simulink model "Channel"  (R2023b)
settings: Solver=VariableStepAuto  StartTime=0.0  StopTime=0.01  MaxStep=1e-3  RelTol=1e-3
libraries: simulink x6, dspsrcs4 x1, dspsigops x1
(part 2 of 3)

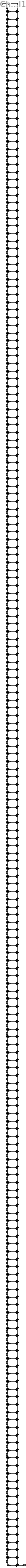
== system Channel/Digital Telecom Project Channel1 ==
  Input : Inport
  BodyDelay{3..205} (203 alike) : Delay  DelayLength=1  InitialCondition=0
  BodyDelay2 : Delay  DelayLength=1  InitialCondition=0  SampleTime=1e-5
  BodyLSum{2..205} (204 alike) : Sum  Inputs=++|  RndMeth=Nearest  SaturateOnIntegerOverflow=on  OutDataTypeStr=Inherit: Same as first input
  b(1) : Gain  Gain=-7.23177798125752776e-05  ParamDataTypeStr=double  RndMeth=Nearest  SaturateOnIntegerOverflow=on  OutDataTypeStr=Inherit: Same as input
  b(10) : Gain  Gain=-0.00017738558129430735  ParamDataTypeStr=double  RndMeth=Nearest  SaturateOnIntegerOverflow=on  OutDataTypeStr=Inherit: Same as input
  b(100) : Gain  Gain=0.0554462164918697528  ParamDataTypeStr=double  RndMeth=Nearest  SaturateOnIntegerOverflow=on  OutDataTypeStr=Inherit: Same as input
  b(101) : Gain  Gain=0.0571275400140215384  ParamDataTypeStr=double  RndMeth=Nearest  SaturateOnIntegerOverflow=on  OutDataTypeStr=Inherit: Same as input
  b(102) : Gain  Gain=0.0581515970344804387  ParamDataTypeStr=double  RndMeth=Nearest  SaturateOnIntegerOverflow=on  OutDataTypeStr=Inherit: Same as input
  b(103) : Gain  Gain=0.0584955166074403385  ParamDataTypeStr=double  RndMeth=Nearest  SaturateOnIntegerOverflow=on  OutDataTypeStr=Inherit: Same as input
  b(104) : Gain  Gain=0.0581515970344804387  ParamDataTypeStr=double  RndMeth=Nearest  SaturateOnIntegerOverflow=on  OutDataTypeStr=Inherit: Same as input
  b(105) : Gain  Gain=0.0571275400140215384  ParamDataTypeStr=double  RndMeth=Nearest  SaturateOnIntegerOverflow=on  OutDataTypeStr=Inherit: Same as input
  b(106) : Gain  Gain=0.0554462164918697528  ParamDataTypeStr=double  RndMeth=Nearest  SaturateOnIntegerOverflow=on  OutDataTypeStr=Inherit: Same as input
  b(107) : Gain  Gain=0.0531450506077565596  ParamDataTypeStr=double  RndMeth=Nearest  SaturateOnIntegerOverflow=on  OutDataTypeStr=Inherit: Same as input
  b(108) : Gain  Gain=0.0502749556371871673  ParamDataTypeStr=double  RndMeth=Nearest  SaturateOnIntegerOverflow=on  OutDataTypeStr=Inherit: Same as input
  b(109) : Gain  Gain=0.0468989161408221791  ParamDataTypeStr=double  RndMeth=Nearest  SaturateOnIntegerOverflow=on  OutDataTypeStr=Inherit: Same as input
  b(11) : Gain  Gain=-0.000177051579349915897  ParamDataTypeStr=double  RndMeth=Nearest  SaturateOnIntegerOverflow=on  OutDataTypeStr=Inherit: Same as input
  b(110) : Gain  Gain=0.0430902630450007082  ParamDataTypeStr=double  RndMeth=Nearest  SaturateOnIntegerOverflow=on  OutDataTypeStr=Inherit: Same as input
  b(111) : Gain  Gain=0.0389306336151945542  ParamDataTypeStr=double  RndMeth=Nearest  SaturateOnIntegerOverflow=on  OutDataTypeStr=Inherit: Same as input
  b(112) : Gain  Gain=0.0345077911752375982  ParamDataTypeStr=double  RndMeth=Nearest  SaturateOnIntegerOverflow=on  OutDataTypeStr=Inherit: Same as input
  b(113) : Gain  Gain=0.0299132143727797242  ParamDataTypeStr=double  RndMeth=Nearest  SaturateOnIntegerOverflow=on  OutDataTypeStr=Inherit: Same as input
  b(114) : Gain  Gain=0.0252397131561066974  ParamDataTypeStr=double  RndMeth=Nearest  SaturateOnIntegerOverflow=on  OutDataTypeStr=Inherit: Same as input
  b(115) : Gain  Gain=0.0205790082061454542  ParamDataTypeStr=double  RndMeth=Nearest  SaturateOnIntegerOverflow=on  OutDataTypeStr=Inherit: Same as input
  b(116) : Gain  Gain=0.0160193674560601164  ParamDataTypeStr=double  RndMeth=Nearest  SaturateOnIntegerOverflow=on  OutDataTypeStr=Inherit: Same as input
  b(117) : Gain  Gain=0.0116434548299792617  ParamDataTypeStr=double  RndMeth=Nearest  SaturateOnIntegerOverflow=on  OutDataTypeStr=Inherit: Same as input
  b(118) : Gain  Gain=0.00752634851574156966  ParamDataTypeStr=double  RndMeth=Nearest  SaturateOnIntegerOverflow=on  OutDataTypeStr=Inherit: Same as input
  b(119) : Gain  Gain=0.00373382597310942688  ParamDataTypeStr=double  RndMeth=Nearest  SaturateOnIntegerOverflow=on  OutDataTypeStr=Inherit: Same as input
  b(12) : Gain  Gain=-0.000168739961757526319  ParamDataTypeStr=double  RndMeth=Nearest  SaturateOnIntegerOverflow=on  OutDataTypeStr=Inherit: Same as input
  b(120) : Gain  Gain=0.000320989051272210042  ParamDataTypeStr=double  RndMeth=Nearest  SaturateOnIntegerOverflow=on  OutDataTypeStr=Inherit: Same as input
  b(121) : Gain  Gain=-0.00266877426121234392  ParamDataTypeStr=double  RndMeth=Nearest  SaturateOnIntegerOverflow=on  OutDataTypeStr=Inherit: Same as input
  b(122) : Gain  Gain=-0.0052044834437449403  ParamDataTypeStr=double  RndMeth=Nearest  SaturateOnIntegerOverflow=on  OutDataTypeStr=Inherit: Same as input
  b(123) : Gain  Gain=-0.00726784415471931015  ParamDataTypeStr=double  RndMeth=Nearest  SaturateOnIntegerOverflow=on  OutDataTypeStr=Inherit: Same as input
  b(124) : Gain  Gain=-0.00885315242129840196  ParamDataTypeStr=double  RndMeth=Nearest  SaturateOnIntegerOverflow=on  OutDataTypeStr=Inherit: Same as input
  b(125) : Gain  Gain=-0.00996687455632458419  ParamDataTypeStr=double  RndMeth=Nearest  SaturateOnIntegerOverflow=on  OutDataTypeStr=Inherit: Same as input
  b(126) : Gain  Gain=-0.0106268662594531452  ParamDataTypeStr=double  RndMeth=Nearest  SaturateOnIntegerOverflow=on  OutDataTypeStr=Inherit: Same as input
  b(127) : Gain  Gain=-0.0108612686273331423  ParamDataTypeStr=double  RndMeth=Nearest  SaturateOnIntegerOverflow=on  OutDataTypeStr=Inherit: Same as input
  b(128) : Gain  Gain=-0.0107072043496892529  ParamDataTypeStr=double  RndMeth=Nearest  SaturateOnIntegerOverflow=on  OutDataTypeStr=Inherit: Same as input
  b(129) : Gain  Gain=-0.010209223554266152  ParamDataTypeStr=double  RndMeth=Nearest  SaturateOnIntegerOverflow=on  OutDataTypeStr=Inherit: Same as input
  b(13) : Gain  Gain=-0.000151261221409517105  ParamDataTypeStr=double  RndMeth=Nearest  SaturateOnIntegerOverflow=on  OutDataTypeStr=Inherit: Same as input
  b(130) : Gain  Gain=-0.00941764136546740724  ParamDataTypeStr=double  RndMeth=Nearest  SaturateOnIntegerOverflow=on  OutDataTypeStr=Inherit: Same as input
  b(131) : Gain  Gain=-0.00838675364453387445  ParamDataTypeStr=double  RndMeth=Nearest  SaturateOnIntegerOverflow=on  OutDataTypeStr=Inherit: Same as input
  b(132) : Gain  Gain=-0.00717304188064623281  ParamDataTypeStr=double  RndMeth=Nearest  SaturateOnIntegerOverflow=on  OutDataTypeStr=Inherit: Same as input
  b(133) : Gain  Gain=-0.00583342353290126295  ParamDataTypeStr=double  RndMeth=Nearest  SaturateOnIntegerOverflow=on  OutDataTypeStr=Inherit: Same as input
  b(134) : Gain  Gain=-0.00442355638748025484  ParamDataTypeStr=double  RndMeth=Nearest  SaturateOnIntegerOverflow=on  OutDataTypeStr=Inherit: Same as input
  b(135) : Gain  Gain=-0.00299629918090278235  ParamDataTypeStr=double  RndMeth=Nearest  SaturateOnIntegerOverflow=on  OutDataTypeStr=Inherit: Same as input
  b(136) : Gain  Gain=-0.00160033930293999416  ParamDataTypeStr=double  RndMeth=Nearest  SaturateOnIntegerOverflow=on  OutDataTypeStr=Inherit: Same as input
  b(137) : Gain  Gain=-0.000279040136813581661  ParamDataTypeStr=double  RndMeth=Nearest  SaturateOnIntegerOverflow=on  OutDataTypeStr=Inherit: Same as input
  b(138) : Gain  Gain=0.000930470592814828992  ParamDataTypeStr=double  RndMeth=Nearest  SaturateOnIntegerOverflow=on  OutDataTypeStr=Inherit: Same as input
  b(139) : Gain  Gain=0.00199799417392200777  ParamDataTypeStr=double  RndMeth=Nearest  SaturateOnIntegerOverflow=on  OutDataTypeStr=Inherit: Same as input
  b(14) : Gain  Gain=-0.000123700880332209607  ParamDataTypeStr=double  RndMeth=Nearest  SaturateOnIntegerOverflow=on  OutDataTypeStr=Inherit: Same as input
  b(140) : Gain  Gain=0.00290061614918906861  ParamDataTypeStr=double  RndMeth=Nearest  SaturateOnIntegerOverflow=on  OutDataTypeStr=Inherit: Same as input
  b(141) : Gain  Gain=0.00362291163889403829  ParamDataTypeStr=double  RndMeth=Nearest  SaturateOnIntegerOverflow=on  OutDataTypeStr=Inherit: Same as input
  b(142) : Gain  Gain=0.00415674988434175472  ParamDataTypeStr=double  RndMeth=Nearest  SaturateOnIntegerOverflow=on  OutDataTypeStr=Inherit: Same as input
  b(143) : Gain  Gain=0.00450106275680541967  ParamDataTypeStr=double  RndMeth=Nearest  SaturateOnIntegerOverflow=on  OutDataTypeStr=Inherit: Same as input
  b(144) : Gain  Gain=0.00466122082854022492  ParamDataTypeStr=double  RndMeth=Nearest  SaturateOnIntegerOverflow=on  OutDataTypeStr=Inherit: Same as input
  b(145) : Gain  Gain=0.0046483380224322246  ParamDataTypeStr=double  RndMeth=Nearest  SaturateOnIntegerOverflow=on  OutDataTypeStr=Inherit: Same as input
  b(146) : Gain  Gain=0.00447847205219086344  ParamDataTypeStr=double  RndMeth=Nearest  SaturateOnIntegerOverflow=on  OutDataTypeStr=Inherit: Same as input
  b(147) : Gain  Gain=0.00417157458074476992  ParamDataTypeStr=double  RndMeth=Nearest  SaturateOnIntegerOverflow=on  OutDataTypeStr=Inherit: Same as input
  b(148) : Gain  Gain=0.00375056466831552712  ParamDataTypeStr=double  RndMeth=Nearest  SaturateOnIntegerOverflow=on  OutDataTypeStr=Inherit: Same as input
  b(149) : Gain  Gain=0.00324026871600793147  ParamDataTypeStr=double  RndMeth=Nearest  SaturateOnIntegerOverflow=on  OutDataTypeStr=Inherit: Same as input
  b(15) : Gain  Gain=-8.54682194051500699e-05  ParamDataTypeStr=double  RndMeth=Nearest  SaturateOnIntegerOverflow=on  OutDataTypeStr=Inherit: Same as input
  b(150) : Gain  Gain=0.00266638467423394813  ParamDataTypeStr=double  RndMeth=Nearest  SaturateOnIntegerOverflow=on  OutDataTypeStr=Inherit: Same as input
  b(151) : Gain  Gain=0.00205451241632236036  ParamDataTypeStr=double  RndMeth=Nearest  SaturateOnIntegerOverflow=on  OutDataTypeStr=Inherit: Same as input
  b(152) : Gain  Gain=0.00142931343546074253  ParamDataTypeStr=double  RndMeth=Nearest  SaturateOnIntegerOverflow=on  OutDataTypeStr=Inherit: Same as input
  b(153) : Gain  Gain=0.000813680276176603399  ParamDataTypeStr=double  RndMeth=Nearest  SaturateOnIntegerOverflow=on  OutDataTypeStr=Inherit: Same as input
  b(154) : Gain  Gain=0.000228095542997559098  ParamDataTypeStr=double  RndMeth=Nearest  SaturateOnIntegerOverflow=on  OutDataTypeStr=Inherit: Same as input
  b(155) : Gain  Gain=-0.00030987781000665378  ParamDataTypeStr=double  RndMeth=Nearest  SaturateOnIntegerOverflow=on  OutDataTypeStr=Inherit: Same as input
  b(156) : Gain  Gain=-0.000785947000839479584  ParamDataTypeStr=double  RndMeth=Nearest  SaturateOnIntegerOverflow=on  OutDataTypeStr=Inherit: Same as input
  b(157) : Gain  Gain=-0.00118935025437075822  ParamDataTypeStr=double  RndMeth=Nearest  SaturateOnIntegerOverflow=on  OutDataTypeStr=Inherit: Same as input
  b(158) : Gain  Gain=-0.00151288960584905225  ParamDataTypeStr=double  RndMeth=Nearest  SaturateOnIntegerOverflow=on  OutDataTypeStr=Inherit: Same as input
  b(159) : Gain  Gain=-0.00175289836764415895  ParamDataTypeStr=double  RndMeth=Nearest  SaturateOnIntegerOverflow=on  OutDataTypeStr=Inherit: Same as input
  b(16) : Gain  Gain=-3.64024111983535668e-05  ParamDataTypeStr=double  RndMeth=Nearest  SaturateOnIntegerOverflow=on  OutDataTypeStr=Inherit: Same as input
  b(160) : Gain  Gain=-0.00190901435619303134  ParamDataTypeStr=double  RndMeth=Nearest  SaturateOnIntegerOverflow=on  OutDataTypeStr=Inherit: Same as input
  b(161) : Gain  Gain=-0.00198393830979729955  ParamDataTypeStr=double  RndMeth=Nearest  SaturateOnIntegerOverflow=on  OutDataTypeStr=Inherit: Same as input
  b(162) : Gain  Gain=-0.0019830220113377095  ParamDataTypeStr=double  RndMeth=Nearest  SaturateOnIntegerOverflow=on  OutDataTypeStr=Inherit: Same as input
  b(163) : Gain  Gain=-0.00191384312739482899  ParamDataTypeStr=double  RndMeth=Nearest  SaturateOnIntegerOverflow=on  OutDataTypeStr=Inherit: Same as input
  b(164) : Gain  Gain=-0.0017856870103015619  ParamDataTypeStr=double  RndMeth=Nearest  SaturateOnIntegerOverflow=on  OutDataTypeStr=Inherit: Same as input
  b(165) : Gain  Gain=-0.00160908251881236499  ParamDataTypeStr=double  RndMeth=Nearest  SaturateOnIntegerOverflow=on  OutDataTypeStr=Inherit: Same as input
  b(166) : Gain  Gain=-0.00139525407679599953  ParamDataTypeStr=double  RndMeth=Nearest  SaturateOnIntegerOverflow=on  OutDataTypeStr=Inherit: Same as input
  b(167) : Gain  Gain=-0.0011556860905953942  ParamDataTypeStr=double  RndMeth=Nearest  SaturateOnIntegerOverflow=on  OutDataTypeStr=Inherit: Same as input
  b(168) : Gain  Gain=-0.000901594504481856383  ParamDataTypeStr=double  RndMeth=Nearest  SaturateOnIntegerOverflow=on  OutDataTypeStr=Inherit: Same as input
  b(169) : Gain  Gain=-0.00064362330173366514  ParamDataTypeStr=double  RndMeth=Nearest  SaturateOnIntegerOverflow=on  OutDataTypeStr=Inherit: Same as input
  b(17) : Gain  Gain=2.31923394344142452e-05  ParamDataTypeStr=double  RndMeth=Nearest  SaturateOnIntegerOverflow=on  OutDataTypeStr=Inherit: Same as input
  b(170) : Gain  Gain=-0.000391395537120529696  ParamDataTypeStr=double  RndMeth=Nearest  SaturateOnIntegerOverflow=on  OutDataTypeStr=Inherit: Same as input
  b(171) : Gain  Gain=-0.000153395226399809535  ParamDataTypeStr=double  RndMeth=Nearest  SaturateOnIntegerOverflow=on  OutDataTypeStr=Inherit: Same as input
  b(172) : Gain  Gain=6.34202859813084985e-05  ParamDataTypeStr=double  RndMeth=Nearest  SaturateOnIntegerOverflow=on  OutDataTypeStr=Inherit: Same as input
  b(173) : Gain  Gain=0.000253526896158335485  ParamDataTypeStr=double  RndMeth=Nearest  SaturateOnIntegerOverflow=on  OutDataTypeStr=Inherit: Same as input
  b(174) : Gain  Gain=0.000413062604855477455  ParamDataTypeStr=double  RndMeth=Nearest  SaturateOnIntegerOverflow=on  OutDataTypeStr=Inherit: Same as input
  b(175) : Gain  Gain=0.000539780548304295751  ParamDataTypeStr=double  RndMeth=Nearest  SaturateOnIntegerOverflow=on  OutDataTypeStr=Inherit: Same as input
  b(176) : Gain  Gain=0.000632725544174888958  ParamDataTypeStr=double  RndMeth=Nearest  SaturateOnIntegerOverflow=on  OutDataTypeStr=Inherit: Same as input
  b(177) : Gain  Gain=0.000692596775144299192  ParamDataTypeStr=double  RndMeth=Nearest  SaturateOnIntegerOverflow=on  OutDataTypeStr=Inherit: Same as input
  b(178) : Gain  Gain=0.000721061107037532863  ParamDataTypeStr=double  RndMeth=Nearest  SaturateOnIntegerOverflow=on  OutDataTypeStr=Inherit: Same as input
  b(179) : Gain  Gain=0.000720840973163188099  ParamDataTypeStr=double  RndMeth=Nearest  SaturateOnIntegerOverflow=on  OutDataTypeStr=Inherit: Same as input
  b(18) : Gain  Gain=9.24341903313585735e-05  ParamDataTypeStr=double  RndMeth=Nearest  SaturateOnIntegerOverflow=on  OutDataTypeStr=Inherit: Same as input
  b(180) : Gain  Gain=0.000695459289895121631  ParamDataTypeStr=double  RndMeth=Nearest  SaturateOnIntegerOverflow=on  OutDataTypeStr=Inherit: Same as input
  b(181) : Gain  Gain=0.000649012321662908792  ParamDataTypeStr=double  RndMeth=Nearest  SaturateOnIntegerOverflow=on  OutDataTypeStr=Inherit: Same as input
  b(182) : Gain  Gain=0.000585821539977197004  ParamDataTypeStr=double  RndMeth=Nearest  SaturateOnIntegerOverflow=on  OutDataTypeStr=Inherit: Same as input
  b(183) : Gain  Gain=0.000510378898786441131  ParamDataTypeStr=double  RndMeth=Nearest  SaturateOnIntegerOverflow=on  OutDataTypeStr=Inherit: Same as input
  b(184) : Gain  Gain=0.000427099839253728482  ParamDataTypeStr=double  RndMeth=Nearest  SaturateOnIntegerOverflow=on  OutDataTypeStr=Inherit: Same as input
  b(185) : Gain  Gain=0.000340170874080033333  ParamDataTypeStr=double  RndMeth=Nearest  SaturateOnIntegerOverflow=on  OutDataTypeStr=Inherit: Same as input
  b(186) : Gain  Gain=0.000253332426038994224  ParamDataTypeStr=double  RndMeth=Nearest  SaturateOnIntegerOverflow=on  OutDataTypeStr=Inherit: Same as input
  b(187) : Gain  Gain=0.000169856054824464949  ParamDataTypeStr=double  RndMeth=Nearest  SaturateOnIntegerOverflow=on  OutDataTypeStr=Inherit: Same as input
  b(188) : Gain  Gain=9.24341903313585735e-05  ParamDataTypeStr=double  RndMeth=Nearest  SaturateOnIntegerOverflow=on  OutDataTypeStr=Inherit: Same as input
  b(189) : Gain  Gain=2.31923394344142452e-05  ParamDataTypeStr=double  RndMeth=Nearest  SaturateOnIntegerOverflow=on  OutDataTypeStr=Inherit: Same as input
  b(19) : Gain  Gain=0.000169856054824464949  ParamDataTypeStr=double  RndMeth=Nearest  SaturateOnIntegerOverflow=on  OutDataTypeStr=Inherit: Same as input
  b(190) : Gain  Gain=-3.64024111983535668e-05  ParamDataTypeStr=double  RndMeth=Nearest  SaturateOnIntegerOverflow=on  OutDataTypeStr=Inherit: Same as input
  b(191) : Gain  Gain=-8.54682194051500699e-05  ParamDataTypeStr=double  RndMeth=Nearest  SaturateOnIntegerOverflow=on  OutDataTypeStr=Inherit: Same as input
  b(192) : Gain  Gain=-0.000123700880332209607  ParamDataTypeStr=double  RndMeth=Nearest  SaturateOnIntegerOverflow=on  OutDataTypeStr=Inherit: Same as input
  b(193) : Gain  Gain=-0.000151261221409517105  ParamDataTypeStr=double  RndMeth=Nearest  SaturateOnIntegerOverflow=on  OutDataTypeStr=Inherit: Same as input
  b(194) : Gain  Gain=-0.000168739961757526319  ParamDataTypeStr=double  RndMeth=Nearest  SaturateOnIntegerOverflow=on  OutDataTypeStr=Inherit: Same as input
  b(195) : Gain  Gain=-0.000177051579349915897  ParamDataTypeStr=double  RndMeth=Nearest  SaturateOnIntegerOverflow=on  OutDataTypeStr=Inherit: Same as input
  b(196) : Gain  Gain=-0.00017738558129430735  ParamDataTypeStr=double  RndMeth=Nearest  SaturateOnIntegerOverflow=on  OutDataTypeStr=Inherit: Same as input
  b(197) : Gain  Gain=-0.000171076363923498202  ParamDataTypeStr=double  RndMeth=Nearest  SaturateOnIntegerOverflow=on  OutDataTypeStr=Inherit: Same as input
  b(198) : Gain  Gain=-0.000159555392738863213  ParamDataTypeStr=double  RndMeth=Nearest  SaturateOnIntegerOverflow=on  OutDataTypeStr=Inherit: Same as input
  b(199) : Gain  Gain=-0.000144225432374725184  ParamDataTypeStr=double  RndMeth=Nearest  SaturateOnIntegerOverflow=on  OutDataTypeStr=Inherit: Same as input
  b(2) : Gain  Gain=-5.2918089340441448e-05  ParamDataTypeStr=double  RndMeth=Nearest  SaturateOnIntegerOverflow=on  OutDataTypeStr=Inherit: Same as input
  b(20) : Gain  Gain=0.000253332426038994224  ParamDataTypeStr=double  RndMeth=Nearest  SaturateOnIntegerOverflow=on  OutDataTypeStr=Inherit: Same as input
  b(200) : Gain  Gain=-0.000126444544888462608  ParamDataTypeStr=double  RndMeth=Nearest  SaturateOnIntegerOverflow=on  OutDataTypeStr=Inherit: Same as input
  b(201) : Gain  Gain=-0.000107432732718147655  ParamDataTypeStr=double  RndMeth=Nearest  SaturateOnIntegerOverflow=on  OutDataTypeStr=Inherit: Same as input
  b(202) : Gain  Gain=-8.82782913535206119e-05  ParamDataTypeStr=double  RndMeth=Nearest  SaturateOnIntegerOverflow=on  OutDataTypeStr=Inherit: Same as input
  b(203) : Gain  Gain=-6.98686931884627554e-05  ParamDataTypeStr=double  RndMeth=Nearest  SaturateOnIntegerOverflow=on  OutDataTypeStr=Inherit: Same as input
  b(204) : Gain  Gain=-5.2918089340441448e-05  ParamDataTypeStr=double  RndMeth=Nearest  SaturateOnIntegerOverflow=on  OutDataTypeStr=Inherit: Same as input
  b(205) : Gain  Gain=-7.23177798125752776e-05  ParamDataTypeStr=double  RndMeth=Nearest  SaturateOnIntegerOverflow=on  OutDataTypeStr=Inherit: Same as input
  b(21) : Gain  Gain=0.000340170874080033333  ParamDataTypeStr=double  RndMeth=Nearest  SaturateOnIntegerOverflow=on  OutDataTypeStr=Inherit: Same as input
  b(22) : Gain  Gain=0.000427099839253728482  ParamDataTypeStr=double  RndMeth=Nearest  SaturateOnIntegerOverflow=on  OutDataTypeStr=Inherit: Same as input
  b(23) : Gain  Gain=0.000510378898786441131  ParamDataTypeStr=double  RndMeth=Nearest  SaturateOnIntegerOverflow=on  OutDataTypeStr=Inherit: Same as input
  b(24) : Gain  Gain=0.000585821539977197004  ParamDataTypeStr=double  RndMeth=Nearest  SaturateOnIntegerOverflow=on  OutDataTypeStr=Inherit: Same as input
  b(25) : Gain  Gain=0.000649012321662908792  ParamDataTypeStr=double  RndMeth=Nearest  SaturateOnIntegerOverflow=on  OutDataTypeStr=Inherit: Same as input
  b(26) : Gain  Gain=0.000695459289895121631  ParamDataTypeStr=double  RndMeth=Nearest  SaturateOnIntegerOverflow=on  OutDataTypeStr=Inherit: Same as input
  b(27) : Gain  Gain=0.000720840973163188099  ParamDataTypeStr=double  RndMeth=Nearest  SaturateOnIntegerOverflow=on  OutDataTypeStr=Inherit: Same as input
  b(28) : Gain  Gain=0.000721061107037532863  ParamDataTypeStr=double  RndMeth=Nearest  SaturateOnIntegerOverflow=on  OutDataTypeStr=Inherit: Same as input
  b(29) : Gain  Gain=0.000692596775144299192  ParamDataTypeStr=double  RndMeth=Nearest  SaturateOnIntegerOverflow=on  OutDataTypeStr=Inherit: Same as input
  b(3) : Gain  Gain=-6.98686931884627554e-05  ParamDataTypeStr=double  RndMeth=Nearest  SaturateOnIntegerOverflow=on  OutDataTypeStr=Inherit: Same as input
  b(30) : Gain  Gain=0.000632725544174888958  ParamDataTypeStr=double  RndMeth=Nearest  SaturateOnIntegerOverflow=on  OutDataTypeStr=Inherit: Same as input
  b(31) : Gain  Gain=0.000539780548304295751  ParamDataTypeStr=double  RndMeth=Nearest  SaturateOnIntegerOverflow=on  OutDataTypeStr=Inherit: Same as input
  b(32) : Gain  Gain=0.000413062604855477455  ParamDataTypeStr=double  RndMeth=Nearest  SaturateOnIntegerOverflow=on  OutDataTypeStr=Inherit: Same as input
  b(33) : Gain  Gain=0.000253526896158335485  ParamDataTypeStr=double  RndMeth=Nearest  SaturateOnIntegerOverflow=on  OutDataTypeStr=Inherit: Same as input
  b(34) : Gain  Gain=6.34202859813084985e-05  ParamDataTypeStr=double  RndMeth=Nearest  SaturateOnIntegerOverflow=on  OutDataTypeStr=Inherit: Same as input
  b(35) : Gain  Gain=-0.000153395226399809535  ParamDataTypeStr=double  RndMeth=Nearest  SaturateOnIntegerOverflow=on  OutDataTypeStr=Inherit: Same as input
  b(36) : Gain  Gain=-0.000391395537120529696  ParamDataTypeStr=double  RndMeth=Nearest  SaturateOnIntegerOverflow=on  OutDataTypeStr=Inherit: Same as input
  b(37) : Gain  Gain=-0.00064362330173366514  ParamDataTypeStr=double  RndMeth=Nearest  SaturateOnIntegerOverflow=on  OutDataTypeStr=Inherit: Same as input
  b(38) : Gain  Gain=-0.000901594504481856383  ParamDataTypeStr=double  RndMeth=Nearest  SaturateOnIntegerOverflow=on  OutDataTypeStr=Inherit: Same as input
  b(39) : Gain  Gain=-0.0011556860905953942  ParamDataTypeStr=double  RndMeth=Nearest  SaturateOnIntegerOverflow=on  OutDataTypeStr=Inherit: Same as input
  b(4) : Gain  Gain=-8.82782913535206119e-05  ParamDataTypeStr=double  RndMeth=Nearest  SaturateOnIntegerOverflow=on  OutDataTypeStr=Inherit: Same as input
  b(40) : Gain  Gain=-0.00139525407679599953  ParamDataTypeStr=double  RndMeth=Nearest  SaturateOnIntegerOverflow=on  OutDataTypeStr=Inherit: Same as input
  b(41) : Gain  Gain=-0.00160908251881236499  ParamDataTypeStr=double  RndMeth=Nearest  SaturateOnIntegerOverflow=on  OutDataTypeStr=Inherit: Same as input
  b(42) : Gain  Gain=-0.0017856870103015619  ParamDataTypeStr=double  RndMeth=Nearest  SaturateOnIntegerOverflow=on  OutDataTypeStr=Inherit: Same as input
  b(43) : Gain  Gain=-0.00191384312739482899  ParamDataTypeStr=double  RndMeth=Nearest  SaturateOnIntegerOverflow=on  OutDataTypeStr=Inherit: Same as input
  b(44) : Gain  Gain=-0.0019830220113377095  ParamDataTypeStr=double  RndMeth=Nearest  SaturateOnIntegerOverflow=on  OutDataTypeStr=Inherit: Same as input
  b(45) : Gain  Gain=-0.00198393830979729955  ParamDataTypeStr=double  RndMeth=Nearest  SaturateOnIntegerOverflow=on  OutDataTypeStr=Inherit: Same as input
  b(46) : Gain  Gain=-0.00190901435619303134  ParamDataTypeStr=double  RndMeth=Nearest  SaturateOnIntegerOverflow=on  OutDataTypeStr=Inherit: Same as input
  b(47) : Gain  Gain=-0.00175289836764415895  ParamDataTypeStr=double  RndMeth=Nearest  SaturateOnIntegerOverflow=on  OutDataTypeStr=Inherit: Same as input
  b(48) : Gain  Gain=-0.00151288960584905225  ParamDataTypeStr=double  RndMeth=Nearest  SaturateOnIntegerOverflow=on  OutDataTypeStr=Inherit: Same as input
  b(49) : Gain  Gain=-0.00118935025437075822  ParamDataTypeStr=double  RndMeth=Nearest  SaturateOnIntegerOverflow=on  OutDataTypeStr=Inherit: Same as input
  b(5) : Gain  Gain=-0.000107432732718147655  ParamDataTypeStr=double  RndMeth=Nearest  SaturateOnIntegerOverflow=on  OutDataTypeStr=Inherit: Same as input
  b(50) : Gain  Gain=-0.000785947000839479584  ParamDataTypeStr=double  RndMeth=Nearest  SaturateOnIntegerOverflow=on  OutDataTypeStr=Inherit: Same as input
  b(51) : Gain  Gain=-0.00030987781000665378  ParamDataTypeStr=double  RndMeth=Nearest  SaturateOnIntegerOverflow=on  OutDataTypeStr=Inherit: Same as input
  b(52) : Gain  Gain=0.000228095542997559098  ParamDataTypeStr=double  RndMeth=Nearest  SaturateOnIntegerOverflow=on  OutDataTypeStr=Inherit: Same as input
  b(53) : Gain  Gain=0.000813680276176603399  ParamDataTypeStr=double  RndMeth=Nearest  SaturateOnIntegerOverflow=on  OutDataTypeStr=Inherit: Same as input
  b(54) : Gain  Gain=0.00142931343546074253  ParamDataTypeStr=double  RndMeth=Nearest  SaturateOnIntegerOverflow=on  OutDataTypeStr=Inherit: Same as input
  b(55) : Gain  Gain=0.00205451241632236036  ParamDataTypeStr=double  RndMeth=Nearest  SaturateOnIntegerOverflow=on  OutDataTypeStr=Inherit: Same as input
  b(56) : Gain  Gain=0.00266638467423394813  ParamDataTypeStr=double  RndMeth=Nearest  SaturateOnIntegerOverflow=on  OutDataTypeStr=Inherit: Same as input
  b(57) : Gain  Gain=0.00324026871600793147  ParamDataTypeStr=double  RndMeth=Nearest  SaturateOnIntegerOverflow=on  OutDataTypeStr=Inherit: Same as input
  b(58) : Gain  Gain=0.00375056466831552712  ParamDataTypeStr=double  RndMeth=Nearest  SaturateOnIntegerOverflow=on  OutDataTypeStr=Inherit: Same as input
  b(59) : Gain  Gain=0.00417157458074476992  ParamDataTypeStr=double  RndMeth=Nearest  SaturateOnIntegerOverflow=on  OutDataTypeStr=Inherit: Same as input
  b(6) : Gain  Gain=-0.000126444544888462608  ParamDataTypeStr=double  RndMeth=Nearest  SaturateOnIntegerOverflow=on  OutDataTypeStr=Inherit: Same as input
  b(60) : Gain  Gain=0.00447847205219086344  ParamDataTypeStr=double  RndMeth=Nearest  SaturateOnIntegerOverflow=on  OutDataTypeStr=Inherit: Same as input
  b(61) : Gain  Gain=0.0046483380224322246  ParamDataTypeStr=double  RndMeth=Nearest  SaturateOnIntegerOverflow=on  OutDataTypeStr=Inherit: Same as input
  b(62) : Gain  Gain=0.00466122082854022492  ParamDataTypeStr=double  RndMeth=Nearest  SaturateOnIntegerOverflow=on  OutDataTypeStr=Inherit: Same as input
  b(63) : Gain  Gain=0.00450106275680541967  ParamDataTypeStr=double  RndMeth=Nearest  SaturateOnIntegerOverflow=on  OutDataTypeStr=Inherit: Same as input
  b(64) : Gain  Gain=0.00415674988434175472  ParamDataTypeStr=double  RndMeth=Nearest  SaturateOnIntegerOverflow=on  OutDataTypeStr=Inherit: Same as input
  b(65) : Gain  Gain=0.00362291163889403829  ParamDataTypeStr=double  RndMeth=Nearest  SaturateOnIntegerOverflow=on  OutDataTypeStr=Inherit: Same as input
  b(66) : Gain  Gain=0.00290061614918906861  ParamDataTypeStr=double  RndMeth=Nearest  SaturateOnIntegerOverflow=on  OutDataTypeStr=Inherit: Same as input
  b(67) : Gain  Gain=0.00199799417392200777  ParamDataTypeStr=double  RndMeth=Nearest  SaturateOnIntegerOverflow=on  OutDataTypeStr=Inherit: Same as input
  b(68) : Gain  Gain=0.000930470592814828992  ParamDataTypeStr=double  RndMeth=Nearest  SaturateOnIntegerOverflow=on  OutDataTypeStr=Inherit: Same as input
  b(69) : Gain  Gain=-0.000279040136813581661  ParamDataTypeStr=double  RndMeth=Nearest  SaturateOnIntegerOverflow=on  OutDataTypeStr=Inherit: Same as input
  b(7) : Gain  Gain=-0.000144225432374725184  ParamDataTypeStr=double  RndMeth=Nearest  SaturateOnIntegerOverflow=on  OutDataTypeStr=Inherit: Same as input
  b(70) : Gain  Gain=-0.00160033930293999416  ParamDataTypeStr=double  RndMeth=Nearest  SaturateOnIntegerOverflow=on  OutDataTypeStr=Inherit: Same as input
  b(71) : Gain  Gain=-0.00299629918090278235  ParamDataTypeStr=double  RndMeth=Nearest  SaturateOnIntegerOverflow=on  OutDataTypeStr=Inherit: Same as input
  b(72) : Gain  Gain=-0.00442355638748025484  ParamDataTypeStr=double  RndMeth=Nearest  SaturateOnIntegerOverflow=on  OutDataTypeStr=Inherit: Same as input
  b(73) : Gain  Gain=-0.00583342353290126295  ParamDataTypeStr=double  RndMeth=Nearest  SaturateOnIntegerOverflow=on  OutDataTypeStr=Inherit: Same as input
  b(74) : Gain  Gain=-0.00717304188064623281  ParamDataTypeStr=double  RndMeth=Nearest  SaturateOnIntegerOverflow=on  OutDataTypeStr=Inherit: Same as input
  b(75) : Gain  Gain=-0.00838675364453387445  ParamDataTypeStr=double  RndMeth=Nearest  SaturateOnIntegerOverflow=on  OutDataTypeStr=Inherit: Same as input
  b(76) : Gain  Gain=-0.00941764136546740724  ParamDataTypeStr=double  RndMeth=Nearest  SaturateOnIntegerOverflow=on  OutDataTypeStr=Inherit: Same as input
  b(77) : Gain  Gain=-0.010209223554266152  ParamDataTypeStr=double  RndMeth=Nearest  SaturateOnIntegerOverflow=on  OutDataTypeStr=Inherit: Same as input
  b(78) : Gain  Gain=-0.0107072043496892529  ParamDataTypeStr=double  RndMeth=Nearest  SaturateOnIntegerOverflow=on  OutDataTypeStr=Inherit: Same as input
  b(79) : Gain  Gain=-0.0108612686273331423  ParamDataTypeStr=double  RndMeth=Nearest  SaturateOnIntegerOverflow=on  OutDataTypeStr=Inherit: Same as input
  b(8) : Gain  Gain=-0.000159555392738863213  ParamDataTypeStr=double  RndMeth=Nearest  SaturateOnIntegerOverflow=on  OutDataTypeStr=Inherit: Same as input
  b(80) : Gain  Gain=-0.0106268662594531452  ParamDataTypeStr=double  RndMeth=Nearest  SaturateOnIntegerOverflow=on  OutDataTypeStr=Inherit: Same as input
  b(81) : Gain  Gain=-0.00996687455632458419  ParamDataTypeStr=double  RndMeth=Nearest  SaturateOnIntegerOverflow=on  OutDataTypeStr=Inherit: Same as input
  b(82) : Gain  Gain=-0.00885315242129840196  ParamDataTypeStr=double  RndMeth=Nearest  SaturateOnIntegerOverflow=on  OutDataTypeStr=Inherit: Same as input
  b(83) : Gain  Gain=-0.00726784415471931015  ParamDataTypeStr=double  RndMeth=Nearest  SaturateOnIntegerOverflow=on  OutDataTypeStr=Inherit: Same as input
  b(84) : Gain  Gain=-0.0052044834437449403  ParamDataTypeStr=double  RndMeth=Nearest  SaturateOnIntegerOverflow=on  OutDataTypeStr=Inherit: Same as input
  b(85) : Gain  Gain=-0.00266877426121234392  ParamDataTypeStr=double  RndMeth=Nearest  SaturateOnIntegerOverflow=on  OutDataTypeStr=Inherit: Same as input
  b(86) : Gain  Gain=0.000320989051272210042  ParamDataTypeStr=double  RndMeth=Nearest  SaturateOnIntegerOverflow=on  OutDataTypeStr=Inherit: Same as input
  b(87) : Gain  Gain=0.00373382597310942688  ParamDataTypeStr=double  RndMeth=Nearest  SaturateOnIntegerOverflow=on  OutDataTypeStr=Inherit: Same as input
  b(88) : Gain  Gain=0.00752634851574156966  ParamDataTypeStr=double  RndMeth=Nearest  SaturateOnIntegerOverflow=on  OutDataTypeStr=Inherit: Same as input
  b(89) : Gain  Gain=0.0116434548299792617  ParamDataTypeStr=double  RndMeth=Nearest  SaturateOnIntegerOverflow=on  OutDataTypeStr=Inherit: Same as input
  b(9) : Gain  Gain=-0.000171076363923498202  ParamDataTypeStr=double  RndMeth=Nearest  SaturateOnIntegerOverflow=on  OutDataTypeStr=Inherit: Same as input
  b(90) : Gain  Gain=0.0160193674560601164  ParamDataTypeStr=double  RndMeth=Nearest  SaturateOnIntegerOverflow=on  OutDataTypeStr=Inherit: Same as input
  b(91) : Gain  Gain=0.0205790082061454542  ParamDataTypeStr=double  RndMeth=Nearest  SaturateOnIntegerOverflow=on  OutDataTypeStr=Inherit: Same as input
  b(92) : Gain  Gain=0.0252397131561066974  ParamDataTypeStr=double  RndMeth=Nearest  SaturateOnIntegerOverflow=on  OutDataTypeStr=Inherit: Same as input
  b(93) : Gain  Gain=0.0299132143727797242  ParamDataTypeStr=double  RndMeth=Nearest  SaturateOnIntegerOverflow=on  OutDataTypeStr=Inherit: Same as input
  b(94) : Gain  Gain=0.0345077911752375982  ParamDataTypeStr=double  RndMeth=Nearest  SaturateOnIntegerOverflow=on  OutDataTypeStr=Inherit: Same as input
  b(95) : Gain  Gain=0.0389306336151945542  ParamDataTypeStr=double  RndMeth=Nearest  SaturateOnIntegerOverflow=on  OutDataTypeStr=Inherit: Same as input
  b(96) : Gain  Gain=0.0430902630450007082  ParamDataTypeStr=double  RndMeth=Nearest  SaturateOnIntegerOverflow=on  OutDataTypeStr=Inherit: Same as input
  b(97) : Gain  Gain=0.0468989161408221791  ParamDataTypeStr=double  RndMeth=Nearest  SaturateOnIntegerOverflow=on  OutDataTypeStr=Inherit: Same as input
  b(98) : Gain  Gain=0.0502749556371871673  ParamDataTypeStr=double  RndMeth=Nearest  SaturateOnIntegerOverflow=on  OutDataTypeStr=Inherit: Same as input
  b(99) : Gain  Gain=0.0531450506077565596  ParamDataTypeStr=double  RndMeth=Nearest  SaturateOnIntegerOverflow=on  OutDataTypeStr=Inherit: Same as input
  Output : Outport
  wires:
  BodyLSum205/1 -> Output/1
  b(205)/1 -> BodyLSum205/2
  BodyDelay205/1 -> b(205)/1
  BodyLSum204/1 -> BodyLSum205/1
  b(204)/1 -> BodyLSum204/1
  BodyDelay204/1 -> BodyDelay205/1, b(204)/1
  BodyLSum203/1 -> BodyLSum204/2
  b(203)/1 -> BodyLSum203/1
  BodyDelay203/1 -> BodyDelay204/1, b(203)/1
  BodyLSum202/1 -> BodyLSum203/2
  b(202)/1 -> BodyLSum202/1
  BodyDelay202/1 -> BodyDelay203/1, b(202)/1
  BodyLSum201/1 -> BodyLSum202/2
  b(201)/1 -> BodyLSum201/1
  BodyDelay201/1 -> BodyDelay202/1, b(201)/1
  BodyLSum200/1 -> BodyLSum201/2
  b(200)/1 -> BodyLSum200/1
  BodyDelay200/1 -> BodyDelay201/1, b(200)/1
  BodyLSum199/1 -> BodyLSum200/2
  b(199)/1 -> BodyLSum199/1
  BodyDelay199/1 -> BodyDelay200/1, b(199)/1
  BodyLSum198/1 -> BodyLSum199/2
  b(198)/1 -> BodyLSum198/1
  BodyDelay198/1 -> BodyDelay199/1, b(198)/1
  BodyLSum197/1 -> BodyLSum198/2
  b(197)/1 -> BodyLSum197/1
  BodyDelay197/1 -> BodyDelay198/1, b(197)/1
  BodyLSum196/1 -> BodyLSum197/2
  b(196)/1 -> BodyLSum196/1
  BodyDelay196/1 -> BodyDelay197/1, b(196)/1
  BodyLSum195/1 -> BodyLSum196/2
  b(195)/1 -> BodyLSum195/1
  BodyDelay195/1 -> BodyDelay196/1, b(195)/1
  BodyLSum194/1 -> BodyLSum195/2
  b(194)/1 -> BodyLSum194/1
  BodyDelay194/1 -> BodyDelay195/1, b(194)/1
  BodyLSum193/1 -> BodyLSum194/2
  b(193)/1 -> BodyLSum193/1
  BodyDelay193/1 -> BodyDelay194/1, b(193)/1
  BodyLSum192/1 -> BodyLSum193/2
  b(192)/1 -> BodyLSum192/1
  BodyDelay192/1 -> BodyDelay193/1, b(192)/1
  BodyLSum191/1 -> BodyLSum192/2
  b(191)/1 -> BodyLSum191/1
  BodyDelay191/1 -> BodyDelay192/1, b(191)/1
  BodyLSum190/1 -> BodyLSum191/2
  b(190)/1 -> BodyLSum190/1
  BodyDelay190/1 -> BodyDelay191/1, b(190)/1
  BodyLSum189/1 -> BodyLSum190/2
  b(189)/1 -> BodyLSum189/1
  BodyDelay189/1 -> BodyDelay190/1, b(189)/1
  BodyLSum188/1 -> BodyLSum189/2
  b(188)/1 -> BodyLSum188/1
  BodyDelay188/1 -> BodyDelay189/1, b(188)/1
  BodyLSum187/1 -> BodyLSum188/2
  b(187)/1 -> BodyLSum187/1
  BodyDelay187/1 -> BodyDelay188/1, b(187)/1
  BodyLSum186/1 -> BodyLSum187/2
  b(186)/1 -> BodyLSum186/1
  BodyDelay186/1 -> BodyDelay187/1, b(186)/1
  BodyLSum185/1 -> BodyLSum186/2
  b(185)/1 -> BodyLSum185/1
  BodyDelay185/1 -> BodyDelay186/1, b(185)/1
  BodyLSum184/1 -> BodyLSum185/2
  b(184)/1 -> BodyLSum184/1
  BodyDelay184/1 -> BodyDelay185/1, b(184)/1
  BodyLSum183/1 -> BodyLSum184/2
  b(183)/1 -> BodyLSum183/1
  BodyDelay183/1 -> BodyDelay184/1, b(183)/1
  BodyLSum182/1 -> BodyLSum183/2
  b(182)/1 -> BodyLSum182/1
  BodyDelay182/1 -> BodyDelay183/1, b(182)/1
  BodyLSum181/1 -> BodyLSum182/2
  b(181)/1 -> BodyLSum181/1
  BodyDelay181/1 -> BodyDelay182/1, b(181)/1
  BodyLSum180/1 -> BodyLSum181/2
  b(180)/1 -> BodyLSum180/1
  BodyDelay180/1 -> BodyDelay181/1, b(180)/1
  BodyLSum179/1 -> BodyLSum180/2
  b(179)/1 -> BodyLSum179/1
  BodyDelay179/1 -> BodyDelay180/1, b(179)/1
  BodyLSum178/1 -> BodyLSum179/2
  b(178)/1 -> BodyLSum178/1
  BodyDelay178/1 -> BodyDelay179/1, b(178)/1
  BodyLSum177/1 -> BodyLSum178/2
  b(177)/1 -> BodyLSum177/1
  BodyDelay177/1 -> BodyDelay178/1, b(177)/1
  BodyLSum176/1 -> BodyLSum177/2
  b(176)/1 -> BodyLSum176/1
  BodyDelay176/1 -> BodyDelay177/1, b(176)/1
  BodyLSum175/1 -> BodyLSum176/2
  b(175)/1 -> BodyLSum175/1
  BodyDelay175/1 -> BodyDelay176/1, b(175)/1
  BodyLSum174/1 -> BodyLSum175/2
  b(174)/1 -> BodyLSum174/1
  BodyDelay174/1 -> BodyDelay175/1, b(174)/1
  BodyLSum173/1 -> BodyLSum174/2
  b(173)/1 -> BodyLSum173/1
  BodyDelay173/1 -> BodyDelay174/1, b(173)/1
  BodyLSum172/1 -> BodyLSum173/2
  b(172)/1 -> BodyLSum172/1
  BodyDelay172/1 -> BodyDelay173/1, b(172)/1
  BodyLSum171/1 -> BodyLSum172/2
  b(171)/1 -> BodyLSum171/1
  BodyDelay171/1 -> BodyDelay172/1, b(171)/1
  BodyLSum170/1 -> BodyLSum171/2
  b(170)/1 -> BodyLSum170/1
  BodyDelay170/1 -> BodyDelay171/1, b(170)/1
  BodyLSum169/1 -> BodyLSum170/2
  b(169)/1 -> BodyLSum169/1
  BodyDelay169/1 -> BodyDelay170/1, b(169)/1
  BodyLSum168/1 -> BodyLSum169/2
  b(168)/1 -> BodyLSum168/1
  BodyDelay168/1 -> BodyDelay169/1, b(168)/1
  BodyLSum167/1 -> BodyLSum168/2
  b(167)/1 -> BodyLSum167/1
  BodyDelay167/1 -> BodyDelay168/1, b(167)/1
  BodyLSum166/1 -> BodyLSum167/2
  b(166)/1 -> BodyLSum166/1
  BodyDelay166/1 -> BodyDelay167/1, b(166)/1
  BodyLSum165/1 -> BodyLSum166/2
  b(165)/1 -> BodyLSum165/1
  BodyDelay165/1 -> BodyDelay166/1, b(165)/1
  BodyLSum164/1 -> BodyLSum165/2
  b(164)/1 -> BodyLSum164/1
  BodyDelay164/1 -> BodyDelay165/1, b(164)/1
  BodyLSum163/1 -> BodyLSum164/2
  b(163)/1 -> BodyLSum163/1
  BodyDelay163/1 -> BodyDelay164/1, b(163)/1
  BodyLSum162/1 -> BodyLSum163/2
  b(162)/1 -> BodyLSum162/1
  BodyDelay162/1 -> BodyDelay163/1, b(162)/1
  BodyLSum161/1 -> BodyLSum162/2
  b(161)/1 -> BodyLSum161/1
  BodyDelay161/1 -> BodyDelay162/1, b(161)/1
  BodyLSum160/1 -> BodyLSum161/2
  b(160)/1 -> BodyLSum160/1
  BodyDelay160/1 -> BodyDelay161/1, b(160)/1
  BodyLSum159/1 -> BodyLSum160/2
  b(159)/1 -> BodyLSum159/1
  BodyDelay159/1 -> BodyDelay160/1, b(159)/1
  BodyLSum158/1 -> BodyLSum159/2
  b(158)/1 -> BodyLSum158/1
  BodyDelay158/1 -> BodyDelay159/1, b(158)/1
  BodyLSum157/1 -> BodyLSum158/2
  b(157)/1 -> BodyLSum157/1
  BodyDelay157/1 -> BodyDelay158/1, b(157)/1
  BodyLSum156/1 -> BodyLSum157/2
  b(156)/1 -> BodyLSum156/1
  BodyDelay156/1 -> BodyDelay157/1, b(156)/1
  BodyLSum155/1 -> BodyLSum156/2
  b(155)/1 -> BodyLSum155/1
  BodyDelay155/1 -> BodyDelay156/1, b(155)/1
  BodyLSum154/1 -> BodyLSum155/2
  b(154)/1 -> BodyLSum154/1
  BodyDelay154/1 -> BodyDelay155/1, b(154)/1
  BodyLSum153/1 -> BodyLSum154/2
  b(153)/1 -> BodyLSum153/1
  BodyDelay153/1 -> BodyDelay154/1, b(153)/1
  BodyLSum152/1 -> BodyLSum153/2
  b(152)/1 -> BodyLSum152/1
  BodyDelay152/1 -> BodyDelay153/1, b(152)/1
  BodyLSum151/1 -> BodyLSum152/2
  b(151)/1 -> BodyLSum151/1
  BodyDelay151/1 -> BodyDelay152/1, b(151)/1
  BodyLSum150/1 -> BodyLSum151/2
  b(150)/1 -> BodyLSum150/1
  BodyDelay150/1 -> BodyDelay151/1, b(150)/1
  BodyLSum149/1 -> BodyLSum150/2
  b(149)/1 -> BodyLSum149/1
  BodyDelay149/1 -> BodyDelay150/1, b(149)/1
  BodyLSum148/1 -> BodyLSum149/2
  b(148)/1 -> BodyLSum148/1
  BodyDelay148/1 -> BodyDelay149/1, b(148)/1
  BodyLSum147/1 -> BodyLSum148/2
  b(147)/1 -> BodyLSum147/1
  BodyDelay147/1 -> BodyDelay148/1, b(147)/1
  BodyLSum146/1 -> BodyLSum147/2
  b(146)/1 -> BodyLSum146/1
  BodyDelay146/1 -> BodyDelay147/1, b(146)/1
  BodyLSum145/1 -> BodyLSum146/2
  b(145)/1 -> BodyLSum145/1
  BodyDelay145/1 -> BodyDelay146/1, b(145)/1
  BodyLSum144/1 -> BodyLSum145/2
  b(144)/1 -> BodyLSum144/1
  BodyDelay144/1 -> BodyDelay145/1, b(144)/1
  BodyLSum143/1 -> BodyLSum144/2
  b(143)/1 -> BodyLSum143/1
  BodyDelay143/1 -> BodyDelay144/1, b(143)/1
  BodyLSum142/1 -> BodyLSum143/2
  b(142)/1 -> BodyLSum142/1
  BodyDelay142/1 -> BodyDelay143/1, b(142)/1
  BodyLSum141/1 -> BodyLSum142/2
  b(141)/1 -> BodyLSum141/1
  BodyDelay141/1 -> BodyDelay142/1, b(141)/1
  BodyLSum140/1 -> BodyLSum141/2
  b(140)/1 -> BodyLSum140/1
  BodyDelay140/1 -> BodyDelay141/1, b(140)/1
  BodyLSum139/1 -> BodyLSum140/2
  b(139)/1 -> BodyLSum139/1
  BodyDelay139/1 -> BodyDelay140/1, b(139)/1
  BodyLSum138/1 -> BodyLSum139/2
  b(138)/1 -> BodyLSum138/1
  BodyDelay138/1 -> BodyDelay139/1, b(138)/1
  BodyLSum137/1 -> BodyLSum138/2
  b(137)/1 -> BodyLSum137/1
  BodyDelay137/1 -> BodyDelay138/1, b(137)/1
  BodyLSum136/1 -> BodyLSum137/2
  b(136)/1 -> BodyLSum136/1
  BodyDelay136/1 -> BodyDelay137/1, b(136)/1
  BodyLSum135/1 -> BodyLSum136/2
  b(135)/1 -> BodyLSum135/1
  BodyDelay135/1 -> BodyDelay136/1, b(135)/1
  BodyLSum134/1 -> BodyLSum135/2
  b(134)/1 -> BodyLSum134/1
  BodyDelay134/1 -> BodyDelay135/1, b(134)/1
  BodyLSum133/1 -> BodyLSum134/2
  b(133)/1 -> BodyLSum133/1
  BodyDelay133/1 -> BodyDelay134/1, b(133)/1
  BodyLSum132/1 -> BodyLSum133/2
  b(132)/1 -> BodyLSum132/1
  BodyDelay132/1 -> BodyDelay133/1, b(132)/1
  BodyLSum131/1 -> BodyLSum132/2
  b(131)/1 -> BodyLSum131/1
  BodyDelay131/1 -> BodyDelay132/1, b(131)/1
  BodyLSum130/1 -> BodyLSum131/2
  b(130)/1 -> BodyLSum130/1
  BodyDelay130/1 -> BodyDelay131/1, b(130)/1
  BodyLSum129/1 -> BodyLSum130/2
  b(129)/1 -> BodyLSum129/1
  BodyDelay129/1 -> BodyDelay130/1, b(129)/1
  BodyLSum128/1 -> BodyLSum129/2
  b(128)/1 -> BodyLSum128/1
  BodyDelay128/1 -> BodyDelay129/1, b(128)/1
  BodyLSum127/1 -> BodyLSum128/2
  b(127)/1 -> BodyLSum127/1
  BodyDelay127/1 -> BodyDelay128/1, b(127)/1
  BodyLSum126/1 -> BodyLSum127/2
  b(126)/1 -> BodyLSum126/1
  BodyDelay126/1 -> BodyDelay127/1, b(126)/1
  BodyLSum125/1 -> BodyLSum126/2
  b(125)/1 -> BodyLSum125/1
  BodyDelay125/1 -> BodyDelay126/1, b(125)/1
  BodyLSum124/1 -> BodyLSum125/2
  b(124)/1 -> BodyLSum124/1
  BodyDelay124/1 -> BodyDelay125/1, b(124)/1
  BodyLSum123/1 -> BodyLSum124/2
  b(123)/1 -> BodyLSum123/1
  BodyDelay123/1 -> BodyDelay124/1, b(123)/1
  BodyLSum122/1 -> BodyLSum123/2
  b(122)/1 -> BodyLSum122/1
  BodyDelay122/1 -> BodyDelay123/1, b(122)/1
  BodyLSum121/1 -> BodyLSum122/2
  b(121)/1 -> BodyLSum121/1
  BodyDelay121/1 -> BodyDelay122/1, b(121)/1
  BodyLSum120/1 -> BodyLSum121/2
  b(120)/1 -> BodyLSum120/1
  BodyDelay120/1 -> BodyDelay121/1, b(120)/1
  BodyLSum119/1 -> BodyLSum120/2
  b(119)/1 -> BodyLSum119/1
  BodyDelay119/1 -> BodyDelay120/1, b(119)/1
  BodyLSum118/1 -> BodyLSum119/2
  b(118)/1 -> BodyLSum118/1
  BodyDelay118/1 -> BodyDelay119/1, b(118)/1
  BodyLSum117/1 -> BodyLSum118/2
  b(117)/1 -> BodyLSum117/1
  BodyDelay117/1 -> BodyDelay118/1, b(117)/1
  BodyLSum116/1 -> BodyLSum117/2
  b(116)/1 -> BodyLSum116/1
  BodyDelay116/1 -> BodyDelay117/1, b(116)/1
  BodyLSum115/1 -> BodyLSum116/2
  b(115)/1 -> BodyLSum115/1
  BodyDelay115/1 -> BodyDelay116/1, b(115)/1
  BodyLSum114/1 -> BodyLSum115/2
  b(114)/1 -> BodyLSum114/1
  BodyDelay114/1 -> BodyDelay115/1, b(114)/1
  BodyLSum113/1 -> BodyLSum114/2
  b(113)/1 -> BodyLSum113/1
  BodyDelay113/1 -> BodyDelay114/1, b(113)/1
  BodyLSum112/1 -> BodyLSum113/2
  b(112)/1 -> BodyLSum112/1
  BodyDelay112/1 -> BodyDelay113/1, b(112)/1
  BodyLSum111/1 -> BodyLSum112/2
  b(111)/1 -> BodyLSum111/1
  BodyDelay111/1 -> BodyDelay112/1, b(111)/1
  BodyLSum110/1 -> BodyLSum111/2
  b(110)/1 -> BodyLSum110/1
  BodyDelay110/1 -> BodyDelay111/1, b(110)/1
  BodyLSum109/1 -> BodyLSum110/2
  b(109)/1 -> BodyLSum109/1
  BodyDelay109/1 -> BodyDelay110/1, b(109)/1
  BodyLSum108/1 -> BodyLSum109/2
  b(108)/1 -> BodyLSum108/1
  BodyDelay108/1 -> BodyDelay109/1, b(108)/1
  BodyLSum107/1 -> BodyLSum108/2
  b(107)/1 -> BodyLSum107/1
  BodyDelay107/1 -> BodyDelay108/1, b(107)/1
  BodyLSum106/1 -> BodyLSum107/2
  b(106)/1 -> BodyLSum106/1
  BodyDelay106/1 -> BodyDelay107/1, b(106)/1
  BodyLSum105/1 -> BodyLSum106/2
  b(105)/1 -> BodyLSum105/1
  BodyDelay105/1 -> BodyDelay106/1, b(105)/1
  BodyLSum104/1 -> BodyLSum105/2
  b(104)/1 -> BodyLSum104/1
  BodyDelay104/1 -> BodyDelay105/1, b(104)/1
  BodyLSum103/1 -> BodyLSum104/2
  b(103)/1 -> BodyLSum103/1
  BodyDelay103/1 -> BodyDelay104/1, b(103)/1
  BodyLSum102/1 -> BodyLSum103/2
  b(102)/1 -> BodyLSum102/1
  BodyDelay102/1 -> BodyDelay103/1, b(102)/1
  BodyLSum101/1 -> BodyLSum102/2
  b(101)/1 -> BodyLSum101/1
  BodyDelay101/1 -> BodyDelay102/1, b(101)/1
  BodyLSum100/1 -> BodyLSum101/2
  b(100)/1 -> BodyLSum100/1
  BodyDelay100/1 -> BodyDelay101/1, b(100)/1
  BodyLSum99/1 -> BodyLSum100/2
  b(99)/1 -> BodyLSum99/1
  BodyDelay99/1 -> BodyDelay100/1, b(99)/1
  BodyLSum98/1 -> BodyLSum99/2
  b(98)/1 -> BodyLSum98/1
  BodyDelay98/1 -> BodyDelay99/1, b(98)/1
  BodyLSum97/1 -> BodyLSum98/2
  b(97)/1 -> BodyLSum97/1
  BodyDelay97/1 -> BodyDelay98/1, b(97)/1
  BodyLSum96/1 -> BodyLSum97/2
  b(96)/1 -> BodyLSum96/1
  BodyDelay96/1 -> BodyDelay97/1, b(96)/1
  BodyLSum95/1 -> BodyLSum96/2
  b(95)/1 -> BodyLSum95/1
  BodyDelay95/1 -> BodyDelay96/1, b(95)/1
  BodyLSum94/1 -> BodyLSum95/2
  b(94)/1 -> BodyLSum94/1
  BodyDelay94/1 -> BodyDelay95/1, b(94)/1
  BodyLSum93/1 -> BodyLSum94/2
  b(93)/1 -> BodyLSum93/1
  BodyDelay93/1 -> BodyDelay94/1, b(93)/1
  BodyLSum92/1 -> BodyLSum93/2
  b(92)/1 -> BodyLSum92/1
  BodyDelay92/1 -> BodyDelay93/1, b(92)/1
  BodyLSum91/1 -> BodyLSum92/2
  b(91)/1 -> BodyLSum91/1
  BodyDelay91/1 -> BodyDelay92/1, b(91)/1
  BodyLSum90/1 -> BodyLSum91/2
  b(90)/1 -> BodyLSum90/1
  BodyDelay90/1 -> BodyDelay91/1, b(90)/1
  BodyLSum89/1 -> BodyLSum90/2
  b(89)/1 -> BodyLSum89/1
  BodyDelay89/1 -> BodyDelay90/1, b(89)/1
  BodyLSum88/1 -> BodyLSum89/2
  b(88)/1 -> BodyLSum88/1
  BodyDelay88/1 -> BodyDelay89/1, b(88)/1
  BodyLSum87/1 -> BodyLSum88/2
  b(87)/1 -> BodyLSum87/1
  BodyDelay87/1 -> BodyDelay88/1, b(87)/1
  BodyLSum86/1 -> BodyLSum87/2
  b(86)/1 -> BodyLSum86/1
  BodyDelay86/1 -> BodyDelay87/1, b(86)/1
  BodyLSum85/1 -> BodyLSum86/2
  b(85)/1 -> BodyLSum85/1
  BodyDelay85/1 -> BodyDelay86/1, b(85)/1
  BodyLSum84/1 -> BodyLSum85/2
  b(84)/1 -> BodyLSum84/1
  BodyDelay84/1 -> BodyDelay85/1, b(84)/1
  BodyLSum83/1 -> BodyLSum84/2
  b(83)/1 -> BodyLSum83/1
  BodyDelay83/1 -> BodyDelay84/1, b(83)/1
  BodyLSum82/1 -> BodyLSum83/2
  b(82)/1 -> BodyLSum82/1
  BodyDelay82/1 -> BodyDelay83/1, b(82)/1
  BodyLSum81/1 -> BodyLSum82/2
  b(81)/1 -> BodyLSum81/1
  BodyDelay81/1 -> BodyDelay82/1, b(81)/1
  BodyLSum80/1 -> BodyLSum81/2
  b(80)/1 -> BodyLSum80/1
  BodyDelay80/1 -> BodyDelay81/1, b(80)/1
  BodyLSum79/1 -> BodyLSum80/2
  b(79)/1 -> BodyLSum79/1
  BodyDelay79/1 -> BodyDelay80/1, b(79)/1
  BodyLSum78/1 -> BodyLSum79/2
  b(78)/1 -> BodyLSum78/1
  BodyDelay78/1 -> BodyDelay79/1, b(78)/1
  BodyLSum77/1 -> BodyLSum78/2
  b(77)/1 -> BodyLSum77/1
  BodyDelay77/1 -> BodyDelay78/1, b(77)/1
  BodyLSum76/1 -> BodyLSum77/2
  b(76)/1 -> BodyLSum76/1
  BodyDelay76/1 -> BodyDelay77/1, b(76)/1
  BodyLSum75/1 -> BodyLSum76/2
  b(75)/1 -> BodyLSum75/1
  BodyDelay75/1 -> BodyDelay76/1, b(75)/1
  BodyLSum74/1 -> BodyLSum75/2
  b(74)/1 -> BodyLSum74/1
  BodyDelay74/1 -> BodyDelay75/1, b(74)/1
  BodyLSum73/1 -> BodyLSum74/2
  b(73)/1 -> BodyLSum73/1
  BodyDelay73/1 -> BodyDelay74/1, b(73)/1
  BodyLSum72/1 -> BodyLSum73/2
  b(72)/1 -> BodyLSum72/1
  BodyDelay72/1 -> BodyDelay73/1, b(72)/1
  BodyLSum71/1 -> BodyLSum72/2
  b(71)/1 -> BodyLSum71/1
  BodyDelay71/1 -> BodyDelay72/1, b(71)/1
  BodyLSum70/1 -> BodyLSum71/2
  b(70)/1 -> BodyLSum70/1
  BodyDelay70/1 -> BodyDelay71/1, b(70)/1
  BodyLSum69/1 -> BodyLSum70/2
  b(69)/1 -> BodyLSum69/1
  BodyDelay69/1 -> BodyDelay70/1, b(69)/1
  BodyLSum68/1 -> BodyLSum69/2
  b(68)/1 -> BodyLSum68/1
  BodyDelay68/1 -> BodyDelay69/1, b(68)/1
  BodyLSum67/1 -> BodyLSum68/2
  b(67)/1 -> BodyLSum67/1
  BodyDelay67/1 -> BodyDelay68/1, b(67)/1
  BodyLSum66/1 -> BodyLSum67/2
  b(66)/1 -> BodyLSum66/1
  BodyDelay66/1 -> BodyDelay67/1, b(66)/1
  BodyLSum65/1 -> BodyLSum66/2
  b(65)/1 -> BodyLSum65/1
  BodyDelay65/1 -> BodyDelay66/1, b(65)/1
  BodyLSum64/1 -> BodyLSum65/2
  b(64)/1 -> BodyLSum64/1
  BodyDelay64/1 -> BodyDelay65/1, b(64)/1
  BodyLSum63/1 -> BodyLSum64/2
  b(63)/1 -> BodyLSum63/1
  BodyDelay63/1 -> BodyDelay64/1, b(63)/1
  BodyLSum62/1 -> BodyLSum63/2
  b(62)/1 -> BodyLSum62/1
  BodyDelay62/1 -> BodyDelay63/1, b(62)/1
  BodyLSum61/1 -> BodyLSum62/2
  b(61)/1 -> BodyLSum61/1
  BodyDelay61/1 -> BodyDelay62/1, b(61)/1
  BodyLSum60/1 -> BodyLSum61/2
  b(60)/1 -> BodyLSum60/1
  BodyDelay60/1 -> BodyDelay61/1, b(60)/1
  BodyLSum59/1 -> BodyLSum60/2
  b(59)/1 -> BodyLSum59/1
  BodyDelay59/1 -> BodyDelay60/1, b(59)/1
  BodyLSum58/1 -> BodyLSum59/2
  b(58)/1 -> BodyLSum58/1
  BodyDelay58/1 -> BodyDelay59/1, b(58)/1
  BodyLSum57/1 -> BodyLSum58/2
  b(57)/1 -> BodyLSum57/1
  BodyDelay57/1 -> BodyDelay58/1, b(57)/1
  BodyLSum56/1 -> BodyLSum57/2
  b(56)/1 -> BodyLSum56/1
  BodyDelay56/1 -> BodyDelay57/1, b(56)/1
  BodyLSum55/1 -> BodyLSum56/2
  b(55)/1 -> BodyLSum55/1
  BodyDelay55/1 -> BodyDelay56/1, b(55)/1
  BodyLSum54/1 -> BodyLSum55/2
  b(54)/1 -> BodyLSum54/1
  BodyDelay54/1 -> BodyDelay55/1, b(54)/1
  BodyLSum53/1 -> BodyLSum54/2
  b(53)/1 -> BodyLSum53/1
  BodyDelay53/1 -> BodyDelay54/1, b(53)/1
  BodyLSum52/1 -> BodyLSum53/2
  b(52)/1 -> BodyLSum52/1
  BodyDelay52/1 -> BodyDelay53/1, b(52)/1
  BodyLSum51/1 -> BodyLSum52/2
  b(51)/1 -> BodyLSum51/1
  BodyDelay51/1 -> BodyDelay52/1, b(51)/1
  BodyLSum50/1 -> BodyLSum51/2
  b(50)/1 -> BodyLSum50/1
  BodyDelay50/1 -> BodyDelay51/1, b(50)/1
  BodyLSum49/1 -> BodyLSum50/2
  b(49)/1 -> BodyLSum49/1
  BodyDelay49/1 -> BodyDelay50/1, b(49)/1
  BodyLSum48/1 -> BodyLSum49/2
  b(48)/1 -> BodyLSum48/1
  BodyDelay48/1 -> BodyDelay49/1, b(48)/1
  BodyLSum47/1 -> BodyLSum48/2
  b(47)/1 -> BodyLSum47/1
  BodyDelay47/1 -> BodyDelay48/1, b(47)/1
  BodyLSum46/1 -> BodyLSum47/2
  b(46)/1 -> BodyLSum46/1
  BodyDelay46/1 -> BodyDelay47/1, b(46)/1
  BodyLSum45/1 -> BodyLSum46/2
  b(45)/1 -> BodyLSum45/1
  BodyDelay45/1 -> BodyDelay46/1, b(45)/1
  BodyLSum44/1 -> BodyLSum45/2
  b(44)/1 -> BodyLSum44/1
  BodyDelay44/1 -> BodyDelay45/1, b(44)/1
  BodyLSum43/1 -> BodyLSum44/2
  b(43)/1 -> BodyLSum43/1
  BodyDelay43/1 -> BodyDelay44/1, b(43)/1
  BodyLSum42/1 -> BodyLSum43/2
  b(42)/1 -> BodyLSum42/1
  BodyDelay42/1 -> BodyDelay43/1, b(42)/1
  BodyLSum41/1 -> BodyLSum42/2
  b(41)/1 -> BodyLSum41/1
  BodyDelay41/1 -> BodyDelay42/1, b(41)/1
  BodyLSum40/1 -> BodyLSum41/2
  b(40)/1 -> BodyLSum40/1
  BodyDelay40/1 -> BodyDelay41/1, b(40)/1
  BodyLSum39/1 -> BodyLSum40/2
  b(39)/1 -> BodyLSum39/1
  BodyDelay39/1 -> BodyDelay40/1, b(39)/1
  BodyLSum38/1 -> BodyLSum39/2
  b(38)/1 -> BodyLSum38/1
  BodyDelay38/1 -> BodyDelay39/1, b(38)/1
  BodyLSum37/1 -> BodyLSum38/2
  b(37)/1 -> BodyLSum37/1
  BodyDelay37/1 -> BodyDelay38/1, b(37)/1
  BodyLSum36/1 -> BodyLSum37/2
  b(36)/1 -> BodyLSum36/1
  BodyDelay36/1 -> BodyDelay37/1, b(36)/1
  BodyLSum35/1 -> BodyLSum36/2
  b(35)/1 -> BodyLSum35/1
  BodyDelay35/1 -> BodyDelay36/1, b(35)/1
  BodyLSum34/1 -> BodyLSum35/2
  b(34)/1 -> BodyLSum34/1
  BodyDelay34/1 -> BodyDelay35/1, b(34)/1
  BodyLSum33/1 -> BodyLSum34/2
  b(33)/1 -> BodyLSum33/1
  BodyDelay33/1 -> BodyDelay34/1, b(33)/1
  BodyLSum32/1 -> BodyLSum33/2
  b(32)/1 -> BodyLSum32/1
  BodyDelay32/1 -> BodyDelay33/1, b(32)/1
  BodyLSum31/1 -> BodyLSum32/2
  b(31)/1 -> BodyLSum31/1
  BodyDelay31/1 -> BodyDelay32/1, b(31)/1
  BodyLSum30/1 -> BodyLSum31/2
  b(30)/1 -> BodyLSum30/1
  BodyDelay30/1 -> BodyDelay31/1, b(30)/1
  BodyLSum29/1 -> BodyLSum30/2
  b(29)/1 -> BodyLSum29/1
  BodyDelay29/1 -> BodyDelay30/1, b(29)/1
  BodyLSum28/1 -> BodyLSum29/2
  b(28)/1 -> BodyLSum28/1
  BodyDelay28/1 -> BodyDelay29/1, b(28)/1
  BodyLSum27/1 -> BodyLSum28/2
  b(27)/1 -> BodyLSum27/1
  BodyDelay27/1 -> BodyDelay28/1, b(27)/1
  BodyLSum26/1 -> BodyLSum27/2
  b(26)/1 -> BodyLSum26/1
  BodyDelay26/1 -> BodyDelay27/1, b(26)/1
  BodyLSum25/1 -> BodyLSum26/2
  b(25)/1 -> BodyLSum25/1
  BodyDelay25/1 -> BodyDelay26/1, b(25)/1
  BodyLSum24/1 -> BodyLSum25/2
  b(24)/1 -> BodyLSum24/1
  BodyDelay24/1 -> BodyDelay25/1, b(24)/1
  BodyLSum23/1 -> BodyLSum24/2
  b(23)/1 -> BodyLSum23/1
  BodyDelay23/1 -> BodyDelay24/1, b(23)/1
  BodyLSum22/1 -> BodyLSum23/2
  b(22)/1 -> BodyLSum22/1
  BodyDelay22/1 -> BodyDelay23/1, b(22)/1
  BodyLSum21/1 -> BodyLSum22/2
  b(21)/1 -> BodyLSum21/1
  BodyDelay21/1 -> BodyDelay22/1, b(21)/1
  BodyLSum20/1 -> BodyLSum21/2
  b(20)/1 -> BodyLSum20/1
  BodyDelay20/1 -> BodyDelay21/1, b(20)/1
  BodyLSum19/1 -> BodyLSum20/2
  b(19)/1 -> BodyLSum19/1
  BodyDelay19/1 -> BodyDelay20/1, b(19)/1
  BodyLSum18/1 -> BodyLSum19/2
  b(18)/1 -> BodyLSum18/1
  BodyDelay18/1 -> BodyDelay19/1, b(18)/1
  BodyLSum17/1 -> BodyLSum18/2
  b(17)/1 -> BodyLSum17/1
  BodyDelay17/1 -> BodyDelay18/1, b(17)/1
  BodyLSum16/1 -> BodyLSum17/2
  b(16)/1 -> BodyLSum16/1
  BodyDelay16/1 -> BodyDelay17/1, b(16)/1
  BodyLSum15/1 -> BodyLSum16/2
  b(15)/1 -> BodyLSum15/1
  BodyDelay15/1 -> BodyDelay16/1, b(15)/1
  BodyLSum14/1 -> BodyLSum15/2
  b(14)/1 -> BodyLSum14/1
  BodyDelay14/1 -> BodyDelay15/1, b(14)/1
  BodyLSum13/1 -> BodyLSum14/2
  b(13)/1 -> BodyLSum13/1
  BodyDelay13/1 -> BodyDelay14/1, b(13)/1
  BodyLSum12/1 -> BodyLSum13/2
  b(12)/1 -> BodyLSum12/1
  BodyDelay12/1 -> BodyDelay13/1, b(12)/1
  BodyLSum11/1 -> BodyLSum12/2
  b(11)/1 -> BodyLSum11/1
  BodyDelay11/1 -> BodyDelay12/1, b(11)/1
  BodyLSum10/1 -> BodyLSum11/2
  b(10)/1 -> BodyLSum10/1
  BodyDelay10/1 -> BodyDelay11/1, b(10)/1
  BodyLSum9/1 -> BodyLSum10/2
  b(9)/1 -> BodyLSum9/1
  BodyDelay9/1 -> BodyDelay10/1, b(9)/1
  BodyLSum8/1 -> BodyLSum9/2
  b(8)/1 -> BodyLSum8/1
  BodyDelay8/1 -> BodyDelay9/1, b(8)/1
  BodyLSum7/1 -> BodyLSum8/2
  b(7)/1 -> BodyLSum7/1
  BodyDelay7/1 -> BodyDelay8/1, b(7)/1
  BodyLSum6/1 -> BodyLSum7/2
  b(6)/1 -> BodyLSum6/1
  BodyDelay6/1 -> BodyDelay7/1, b(6)/1
  BodyLSum5/1 -> BodyLSum6/2
  b(5)/1 -> BodyLSum5/1
  BodyDelay5/1 -> BodyDelay6/1, b(5)/1
  BodyLSum4/1 -> BodyLSum5/2
  b(4)/1 -> BodyLSum4/1
  BodyDelay4/1 -> BodyDelay5/1, b(4)/1
  BodyLSum3/1 -> BodyLSum4/2
  b(3)/1 -> BodyLSum3/1
  BodyDelay3/1 -> BodyDelay4/1, b(3)/1
  BodyLSum2/1 -> BodyLSum3/2
  b(2)/1 -> BodyLSum2/1
  BodyDelay2/1 -> BodyDelay3/1, b(2)/1
  b(1)/1 -> BodyLSum2/2
  Input/1 -> BodyDelay2/1, b(1)/1
